simulink model "MultirotorModel"  (R2022b)
settings: Solver=VariableStepAuto  StartTime=0.0  StopTime=200  FixedStep=0.005  RelTol=1e-3  EnableMultiTasking=on
undefined symbols (not defined in the file): Controller, decyear, DiscIntNeverNeededParam, DroneMass, Dz, Earth, Gravity, initialConditions, Iz, leapyear, mapmatrix, Nz, Pz, startFlightTime, UAVSampleTime, Vehicle, WGS84
libraries: slpidlib x13, aerolibtransform2 x7, uavalgslib x6, simulink x2, sharedutil x2, aerolibconvert2 x2, sharedTrackingLibrary x2, aerolibatmos2 x1, aerolibgravity2 x1, shared6dof x1, aerolibasang x1, sensorinslib x1
(part 4 of 4)

== matlab function MultirotorModel/Inner Loop and Plant Model/Low-FidelityModel/Position and Acceleration Control/Position Control/MATLAB Function2 ==
  data: pose input; maxlidarrange input; pcrange output; mapmatrix input; pcangle output
function [pcrange, pcangle]  = pcEst(pose,maxlidarrange, mapmatrix)
% x,y,theta should be the real position
% load mapdata.mat mapmatrix

x = pose(1); y = pose(2); theta = pose(3);
pidata_test = linspace(pi,-pi,1084);
pidata_test = pidata_test';
pidata_test = pidata_test(1:end-1,1);
pidata_test(1,1) = -pidata_test(1,1);

pc = lidarScan(mapmatrix);

% figure(1)
% 
% 
% plot(pc.Cartesian(:,1), pc.Cartesian(:,2),'.','MarkerSize',3,'color','m')


new_pc = transformScan(pc, [-x -y 0]);
new_pc = transformScan(new_pc, [0 0 -theta]);
new_pc = new_pc.removeInvalidData;
range = new_pc.Ranges;
angle = new_pc.Angles;
cart = new_pc.Cartesian;
num = length(range);

pcangle = pidata_test;
pcrange = maxlidarrange*ones(length(pidata_test),1);
pcData = lidarScan(pcrange,pcangle);

pidata_test(1,1) = -pidata_test(1,1);
pidata_test = [pidata_test;-pi];

for i = 1:num   % num = 77463
    
    for j = 1:length(pidata_test)-1
        if pidata_test(j+1)<angle(i) && angle(i)<=pidata_test(j)
            if range(i) <= pcrange(j)
            pcrange(j) = range(i);
            end
        end
    end
end

for i = 1: length(pcrange)
    if pcrange(i) == maxlidarrange
        pcrange(i) = NaN;
    end
end

% pcData = lidarScan(pcrange,pcangle);

% % 
% figure(3)
% plot(pcData.Cartesian(:,1),pcData.Cartesian(:,2),'.','MarkerSize',3,'color','m')
% % 
% figure(3)
% plot(new_pc.Cartesian(:,1),new_pc.Cartesian(:,2),'.','MarkerSize',3,'color','m')



end

== matlab function MultirotorModel/Inner Loop and Plant Model/Low-FidelityModel/Position and Acceleration Control/Position Control/MATLAB Function3 ==
  data: u_1 input; u_2 input; index input; u_out output double; xi input
function u_out= safeoutput(u_1,u_2,index,xi)

% u2 = u_2;
% u1 = u_1;
u1 = double(zeros([2,1]));
u2 = double(zeros([2,1]));
u_ast = double(zeros([2,1]));
u_out = double(zeros([3,1]));
u1 = [u_1(1);u_1(2)];
% u1 = u1';
u2 = [u_2(1);u_2(2)];
% u2 = u2';
m = 2;
R = eye(m);
% u_alpha = u1; 
options = optimoptions(@fmincon,'Display','off','Algorithm','sqp',...
    'SpecifyObjectiveGradient',true,'SpecifyConstraintGradient',true);

% constraint_matrix{1} = 2*eye(m);
% constraint_coefficient{1} = [0, 0]';
% constraint_constant{1} = [0, 0]';
% acc_gps1>acc_gps2
constraint_matrix = cell([1,2]);
constraint_matrix1 = cell(1);
constraint_matrix2 = cell(1);
constraint_coefficient =cell([1,2]);
constraint_coefficient1=cell(1);
constraint_coefficient2=cell(1);
constraint_constant = cell([1,2]);
constraint_constant1 = cell(1);
constraint_constant2 = cell(1);
constraint_matrix{1} = 2*eye(m);
constraint_coefficient{1} = -2*u1;
constraint_constant{1} = u1'*u1-xi^2;
constraint_matrix{2} = 2*eye(m);
constraint_coefficient{2} = -2*u1;
constraint_constant{2} = u1'*u1-xi^2;

% constraint_matrix1{1} = 2*eye(m);
% constraint_coefficient1{1} = -2*u1;
% constraint_constant1{1} = u1'*u1-xi^2;
% constraint_matrix2{1} = 2*eye(m);
% constraint_coefficient2{1} = -2*u2;
% constraint_constant2{1} = u2'*u2-xi^2;
% constr_mat = [constraint_matrix1,constraint_matrix2];
% constr_coeff = [constraint_coefficient1, constraint_coefficient1];
% constr_const = [constraint_constant1, constraint_constant2];
% 
% constraint_matrix{1} = constr_mat(1);
% constraint_coefficient{1} = constr_coeff(1);
% constraint_constant{1} = constr_const(1);
% constraint_matrix{2} = constr_mat[2];
% constraint_coefficient{2} = constr_coeff(2);
% constraint_constant{2} = constr_const(2);

fun1 = @(z) quadobj(z,2*R,-2*u1,u1'*u1);
fun2 = @(z) quadobj(z,2*R,-2*u2,u2'*u2);
nonlconstr = @(z) quadconstr(z,constraint_matrix,constraint_coefficient,constraint_constant);
x0 = [0;0]; % column vector
% x0 = start_point;
[u_ast,fval,eflag,output,lambda] = fmincon(fun1,x0,...
    [],[],[],[],[],[],nonlconstr,options);

% u_out = u_ast;
% u_ast = single(u_ast);
if eflag == 1 && index == 3
    u_out = [u_ast', u_1(3)]';

elseif index == 1
    constraint_matrix1{1} = 2*eye(m);
    constraint_coefficient1{1} = -2*u1;
    constraint_constant1{1} = u1'*u1-xi^2;
    nonlconstr = @(z) quadconstr(z,constraint_matrix1,constraint_coefficient1,constraint_constant1);
    [u_ast,fval,eflag,output,lambda] = fmincon(fun1,x0,...
        [],[],[],[],[],[],nonlconstr,options);
%     u_ast = single(u_ast);
    u_out = [u_ast', u_1(3)]';

elseif index == 2
    constraint_matrix2{1} = 2*eye(m);
    constraint_coefficient2{1} = -2*u2;
    constraint_constant2{1} = u2'*u2-xi^2;
    nonlconstr = @(z) quadconstr(z,constraint_matrix2,constraint_coefficient2,constraint_constant2);
    [u_ast,fval,eflag,output,lambda] = fmincon(fun2,x0,...
        [],[],[],[],[],[],nonlconstr,options);
    u_out = [u_ast', u_2(3)]';
%     u_out1 = u_ast(1);
%     u_out2 = u_ast(2);
%     u_out3 = u_2(3);

end

== matlab function MultirotorModel/Inner Loop and Plant Model/Low-FidelityModel/INS6/MATLAB Function ==
  data: truePosition input; position output; trueVelocity input; velocity output; orientation output; trueOrientation input
function [position, velocity, orientation] = simINS(truePosition,trueVelocity,trueOrientation)
gTruth = struct('Position',truePosition,'Velocity',trueVelocity,'Orientation',trueOrientation);
INS = insSensor("PositionAccuracy",0.1,'YawAccuracy',0);
insMeas = INS(gTruth);
position = insMeas.Position;
velocity = insMeas.Velocity;
orientation = insMeas.Orientation;
end

== matlab function MultirotorModel/Inner Loop and Plant Model/Low-FidelityModel/INS2/MATLAB Function ==
  data: truePosition input; position output; trueVelocity input; velocity output; orientation output; trueOrientation input
function [position, velocity, orientation] = simINS(truePosition,trueVelocity,trueOrientation)
gTruth = struct('Position',truePosition,'Velocity',trueVelocity,'Orientation',trueOrientation);
% INS = insSensor("PositionAccuracy",[0.1 0.1 0.1],'RollAccuracy',0,...
%     'PitchAccuracy',0,'VelocityAccuracy',0,'YawAccuracy',0);
INS = insSensor('RollAccuracy',0,'PitchAccuracy',0,'YawAccuracy',0,'PositionAccuracy',[0.001 0.001 0.001],...
    'VelocityAccuracy',0,'AccelerationAccuracy',0);
insMeas = INS(gTruth);
position = insMeas.Position;
velocity = insMeas.Velocity;
orientation = insMeas.Orientation;
end

== matlab function MultirotorModel/Inner Loop and Plant Model/Low-FidelityModel/INS1/MATLAB Function ==
  data: truePosition input; position output; trueVelocity input; velocity output; orientation output; trueOrientation input
function [position, velocity, orientation] = simINS(truePosition,trueVelocity,trueOrientation)
gTruth = struct('Position',truePosition,'Velocity',trueVelocity,'Orientation',trueOrientation);
% INS = insSensor("PositionAccuracy",[0.1 0.1 0.1],'RollAccuracy',0,...
%     'PitchAccuracy',0,'VelocityAccuracy',0,'YawAccuracy',0);
INS = insSensor('RollAccuracy',0,'PitchAccuracy',0,'YawAccuracy',0,'PositionAccuracy',[0.001 0.001 0.001],...
    'VelocityAccuracy',0,'AccelerationAccuracy',0);
insMeas = INS(gTruth);
position = insMeas.Position;
x =  position(1);
y = -position(2);
if y <= 55
    x = x - 20;
end
position(1) = x;
velocity = insMeas.Velocity;
orientation = insMeas.Orientation;
end

== matlab function MultirotorModel/Inner Loop and Plant Model/Low-FidelityModel/Assemble UAV State Bus/Generate GPS Data/Embedded MATLAB Function1 ==
  data: cog output; Vn input; Ve input
function cog = getCOG(Vn, Ve)
% This block supports an embeddable subset of the MATLAB language.
% See the help menu for details. 

cog = atan2(Ve,Vn);
if cog < 0;
    cog = cog + 2*pi;
end

== matlab function MultirotorModel/Inner Loop and Plant Model/High-FidelityModel/Control System/Controller/Position Controller/Position error transformation (Earth to Body frame) ==
  data: yaw input; xy_err_earth input; xy_err_body output
function xy_err_body = LTP2B2D(yaw,xy_err_earth)

transformation = [cos(yaw), sin(yaw); -sin(yaw),  cos(yaw)];
xy_err_body = transformation * xy_err_earth;


end

== matlab function MultirotorModel/Inner Loop and Plant Model/High-FidelityModel/Control System/Controller/Position Controller/Velocity error transformation (Earth to Body frame) ==
  data: yaw input; xy_err_earth input; xy_err_body output
function xy_err_body = LTP2B2D(yaw,xy_err_earth)

transformation = [cos(yaw), sin(yaw); -sin(yaw),  cos(yaw)];
xy_err_body = transformation * xy_err_earth;


end

== stateflow chart MultirotorModel/Guidance Logic/Full Guidance Logic/Guidance Stateflow/Guidance Mode Selector ==
  settings: updateMethod=DISCRETE  sampleTime=UAVSampleTime*4
  state GuidanceLogic
    state OnGround
    state Takeoff
    state WP
    state Orbit
    state Land
      state ToLand
      state Descend
      (default) -> ToLand
      ToLand -> Descend : [norm(Pose(1:2)-ToWP.position(1:2)) <= 2]
    (default) -> OnGround
    OnGround -> (junction 5) : [startFlight==1]
    Takeoff -> WP : [Pose(3) <= -ToWP.position(3)]
    GuidanceLogic -> (junction 5) : [hasChanged(mode)]
    (junction 5) -> Takeoff [order 1] : [mode == 1]
    (junction 5) -> (junction 12) [order 2]
    (junction 12) -> WP [order 1] : [mode==2]
    (junction 12) -> (junction 17) [order 2]
    (junction 17) -> Orbit [order 1] : [mode==3]
    (junction 17) -> (junction 22) [order 2]
    (junction 22) -> Land
    Land -> GuidanceLogic : [Pose(3)>=-0.1]{Status = 2}
  (default) -> GuidanceLogic
  data: sf_internal_action_state_placeholder_data local double size=1 =0; sf_internal_action_state_placeholder_data local double size=1 =0; sf_internal_action_state_placeholder_data local double size=1 =0; sf_internal_action_state_placeholder_data local double size=1 =0; sf_internal_action_state_placeholder_data local double size=1 =0; mode input; ToWP input Bus: uavPathManagerBus; InnerLoopCmds output Bus: innerLoopCmdsBus; Status output uint8; FromWP input Bus: uavPathManagerBus; Pose input; startFlight input
